simulink model "oneparamchange"  (Simulink 6.1)
settings: Solver=ode45  StartTime=0.0  StopTime=10.0  RelTol=1e-3
values from neighbouring files (symbols this model uses):
  sp = 0.002    [Main.m]
undefined symbols (not defined in the file or in its folder): sfunxy_plot
libraries: simulink x1
settings Model: LastModifiedBy=fhuang
settings DebuggingCC: SolverPrmCheckMsg=warning

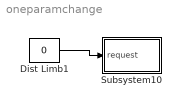
== system oneparamchange ==
  Dist Limb1 : Constant  Value=0
  Subsystem10 : Subsystem
  wires:
  Dist Limb1/1 -> Subsystem10/1(request)

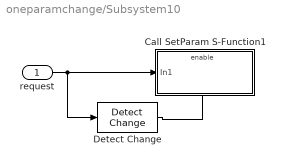
== system oneparamchange/Subsystem10 ==
  request : Inport  Port=1  LatchInput=off
  Call SetParam S-Function1 : Subsystem  TreatAsAtomicUnit=on
  Detect Change : simulink/Logic and Bit Operations/Detect Change  vinit=0
  wires:
  Detect Change/1 -> Call SetParam S-Function1/Enable
  request/1 -> Call SetParam S-Function1/1(In1), Detect Change/1

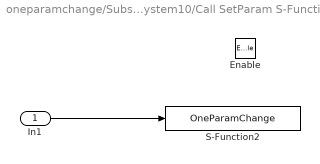
== system oneparamchange/Subsystem10/Call SetParam S-Function1 ==
  In1 : Inport  Port=1  LatchInput=off
  Enable : EnablePort
  S-Function2 : S-Function  StartFcn=sfunxy_plot([],[],[],'Start')  StopFcn=sfunxy_plot([],[],[],'Stop')  FunctionName=OneParamChange  Parameters=sp,'ConstantBlockName'
  wires:
  In1/1 -> S-Function2/1
